simulink model "asynchronous_model"  (R2020a)
settings: Solver=FixedStepAuto  StartTime=0.0  StopTime=50  FixedStep=0.01  MaxStep=.001  RelTol=1e-3
values from neighbouring files (symbols this model uses):
  C_viscous = 0    [load_system_param.m]    (also in run_one_simulation.m = sys_param('C_viscous'); run_simulation.m = sys_param('C_viscous'))
  Gamma = 0.00107    [load_system_param.m]    (also in run_one_simulation.m = sys_param('Gamma'); run_simulation.m = sys_param('Gamma'))
  Inertia = 0.0023    [load_system_param.m]    (also in run_one_simulation.m = sys_param('I'); run_simulation.m = sys_param('I'))
  K = 0.525    [load_system_param.m]    (also in run_one_simulation.m = sys_param('K'); run_simulation.m = sys_param('K'))
  K_muscle = 0    [load_system_param.m]    (also in run_one_simulation.m = sys_param('K_muscle'); run_simulation.m = sys_param('K_muscle'))
  SA_kernel = asynch_gain * gain_constant * (1 - K_r) * temp_kernel    [run_one_simulation.m]    (also in run_simulation.m = asynch_gain * gain_constant * (1 - synch_gain_range(k)) * te)
  synch_gain = K_r * gain_constant    [run_one_simulation.m]    (also in run_simulation.m = synch_gain_range(k) * gain_constant)
  v_initial = 0    [load_system_param.m]    (also in run_one_simulation.m = sys_param('v_initial'); run_simulation.m = sys_param('v_initial'))
  x_initial = 0.1    [load_system_param.m]    (also in run_one_simulation.m = sys_param('x_initial'); run_simulation.m = sys_param('x_initial'))
undefined symbols (not defined in the file or in its folder): synch_w
settings Model: OrderedModelArguments=off  Creator=nickgravish  LastModifiedBy=Administrator
settings DataIOCC: ReturnWorkspaceOutputs=off
settings DebuggingCC: ArithmeticOperatorsInVariantConditions=warning
settings SFSimCC: SimUseLocalCustomCode=off  CustomCodeUndefinedFunction=UseInterfaceOnly
settings RTWCC: RTWUseLocalCustomCode=off
settings CodeAppCC: StateflowObjectComments=on
settings SimscapeCC: SimscapeNormalizeSystem=off

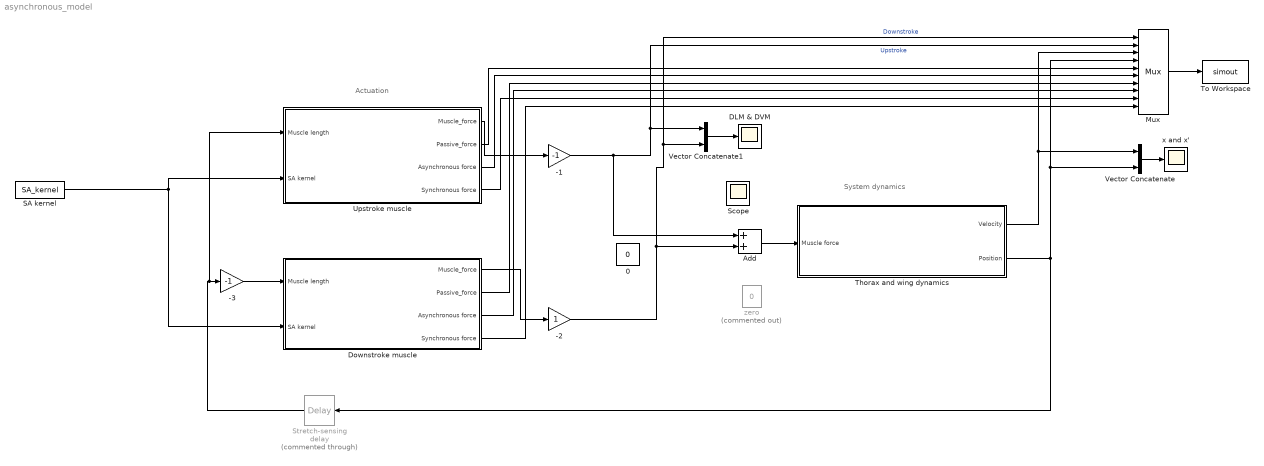
== system asynchronous_model ==
  note: Actuation
  note: System dynamics
  -1 : Gain  Gain=-1
  -2 : Gain
  -3 : Gain  Gain=-1
  Add : Sum
  DLM & DVM : Scope
  Downstroke muscle : Subsystem
  Mux : Mux  Inputs=10
  SA kernel : Constant  Value=SA_kernel
  Stretch-sensing delay : TransportDelay  Commented=through  DelayTime=0
  Thorax and wing dynamics : Subsystem
  To Workspace : ToWorkspace  VariableName=simout  SaveFormat=Timeseries  SampleTime=-1
  Upstroke muscle : Subsystem
  Vector Concatenate : Concatenate
  Vector Concatenate1 : Concatenate
  x and x' : Scope
  zero : Constant  Commented=on  Value=0
  0 : Constant  IOType=siggen  Value=0
  Scope : Scope
  wires:
  Vector Concatenate/1 -> x and x'/1
  -2/1 -> Add/2, Mux/1, Vector Concatenate1/2  "Downstroke"
  -1/1 -> Mux/2, Vector Concatenate1/1, Add/1  "Upstroke"
  Vector Concatenate1/1 -> DLM & DVM/1
  Mux/1 -> To Workspace/1
  Downstroke muscle/1(Muscle_force) -> -2/1
  Thorax and wing dynamics/1(Velocity) -> Mux/3, Vector Concatenate/1
  Thorax and wing dynamics/2(Position) -> Vector Concatenate/2, Mux/4, Stretch-sensing delay/1
  Upstroke muscle/1(Muscle_force) -> -1/1
  Stretch-sensing delay/1 -> Upstroke muscle/1(Muscle length), -3/1
  SA kernel/1 -> Upstroke muscle/2(SA kernel), Downstroke muscle/2(SA kernel)
  -3/1 -> Downstroke muscle/1(Muscle length)
  Downstroke muscle/3(Asynchronous force) -> Mux/8
  Downstroke muscle/2(Passive_force) -> Mux/7
  Upstroke muscle/3(Asynchronous force) -> Mux/6
  Upstroke muscle/2(Passive_force) -> Mux/5
  Add/1 -> Thorax and wing dynamics/1(Muscle force)
  Upstroke muscle/4(Synchronous force) -> Mux/9
  Downstroke muscle/4(Synchronous force) -> Mux/10

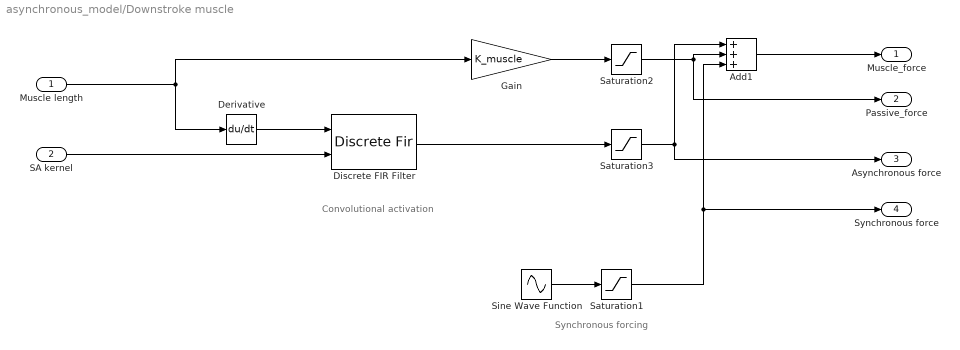
== system asynchronous_model/Downstroke muscle ==
  note: Convolutional activation
  note: Synchronous forcing
  Muscle length : Inport
  SA kernel : Inport  Port=2
  Add1 : Sum  Inputs=+++
  Derivative : Derivative
  Discrete FIR Filter : DiscreteFir  CoefSource=Input port  Coefficients=[0, 0, 2]  InputProcessing=Columns as channels (frame based)
      settings: InputPortMap=u0,u1
  Gain : Gain  Gain=K_muscle
  Saturation1 : Saturate  UpperLimit=Inf  LowerLimit=0
  Saturation2 : Saturate  UpperLimit=Inf  LowerLimit=0
  Saturation3 : Saturate  UpperLimit=Inf  LowerLimit=0
  Sine Wave Function : Sin  Amplitude=synch_gain  Frequency=synch_w  Phase=pi  SampleTime=0
  Muscle_force : Outport
  Passive_force : Outport  Port=2
  Asynchronous force : Outport  Port=3
  Synchronous force : Outport  Port=4
  wires:
  SA kernel/1 -> Discrete FIR Filter/2
  Add1/1 -> Muscle_force/1
  Gain/1 -> Saturation2/1
  Muscle length/1 -> Gain/1, Derivative/1
  Saturation2/1 -> Add1/2, Passive_force/1
  Saturation3/1 -> Add1/1, Asynchronous force/1
  Derivative/1 -> Discrete FIR Filter/1
  Discrete FIR Filter/1 -> Saturation3/1
  Saturation1/1 -> Synchronous force/1, Add1/3
  Sine Wave Function/1 -> Saturation1/1

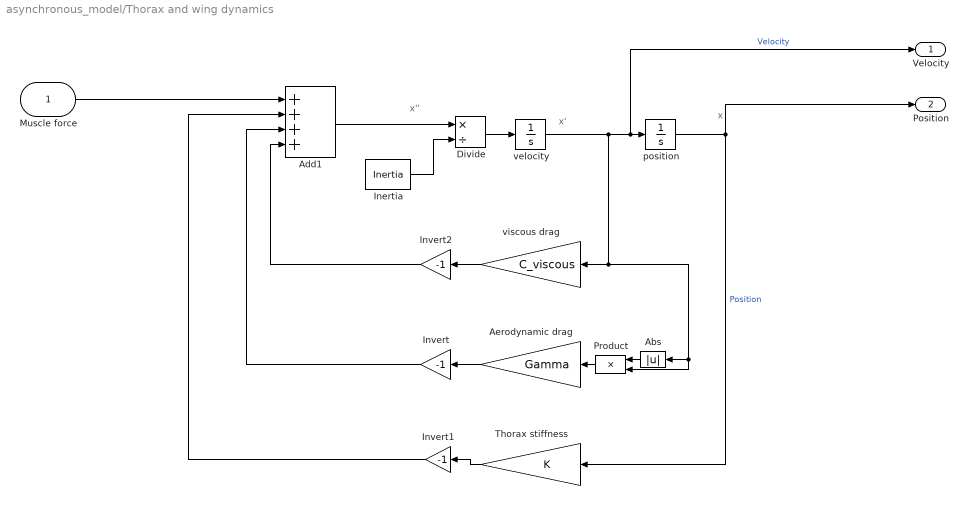
== system asynchronous_model/Thorax and wing dynamics ==
  note: x
  note: x''
  note: x'
  Muscle force : Inport
  Abs : Abs
  Add1 : Sum  Inputs=++++
  Aerodynamic drag : Gain  Gain=Gamma
  Divide : Product  Inputs=*/
  Inertia : Constant  Value=Inertia
  Invert : Gain  Gain=-1
  Invert1 : Gain  Gain=-1
  Invert2 : Gain  Gain=-1
  Product : Product
  Thorax stiffness : Gain  Gain=K
  position : Integrator  InitialCondition=x_initial  ContinuousStateAttributes='Position'
  velocity : Integrator  InitialCondition=v_initial  ContinuousStateAttributes='Velocity'
  viscous drag : Gain  Gain=C_viscous
  Velocity : Outport
  Position : Outport  Port=2
  wires:
  Aerodynamic drag/1 -> Invert/1
  Thorax stiffness/1 -> Invert1/1
  Divide/1 -> velocity/1
  Add1/1 -> Divide/1
  Muscle force/1 -> Add1/1
  velocity/1 -> Product/2, Abs/1, viscous drag/1, Velocity/1, position/1  "Velocity"
  viscous drag/1 -> Invert2/1
  Inertia/1 -> Divide/2
  position/1 -> Thorax stiffness/1, Position/1  "Position"
  Invert2/1 -> Add1/4
  Abs/1 -> Product/1
  Product/1 -> Aerodynamic drag/1
  Invert/1 -> Add1/3
  Invert1/1 -> Add1/2

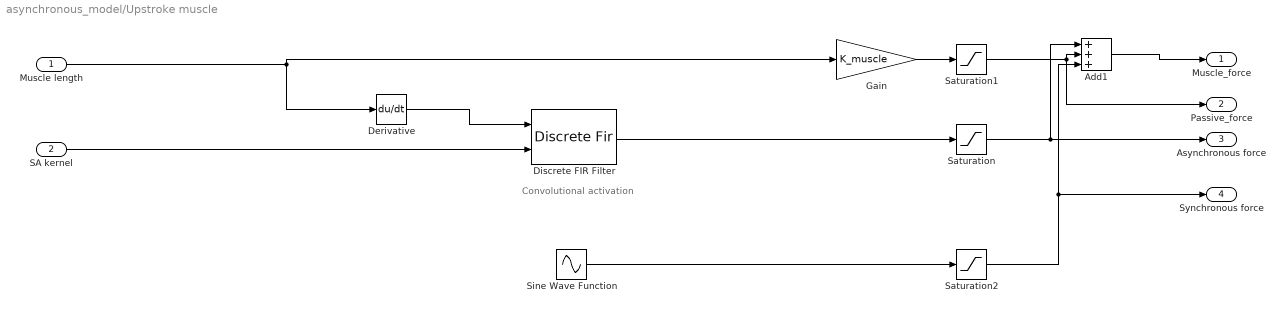
== system asynchronous_model/Upstroke muscle ==
  note: Convolutional activation
  Muscle length : Inport
  SA kernel : Inport  Port=2
  Add1 : Sum  Inputs=+++
  Derivative : Derivative
  Discrete FIR Filter : DiscreteFir  CoefSource=Input port  Coefficients=[0, 0, 2]  InputProcessing=Columns as channels (frame based)
      settings: InputPortMap=u0,u1
  Gain : Gain  Gain=K_muscle
  Saturation : Saturate  UpperLimit=Inf  LowerLimit=0
  Saturation1 : Saturate  UpperLimit=Inf  LowerLimit=0
  Saturation2 : Saturate  UpperLimit=Inf  LowerLimit=0
  Sine Wave Function : Sin  Amplitude=synch_gain  Frequency=synch_w  SampleTime=0
  Muscle_force : Outport
  Passive_force : Outport  Port=2
  Asynchronous force : Outport  Port=3
  Synchronous force : Outport  Port=4
  wires:
  Gain/1 -> Saturation1/1
  Saturation/1 -> Asynchronous force/1, Add1/1
  Muscle length/1 -> Derivative/1, Gain/1
  SA kernel/1 -> Discrete FIR Filter/2
  Add1/1 -> Muscle_force/1
  Saturation1/1 -> Passive_force/1, Add1/2
  Discrete FIR Filter/1 -> Saturation/1
  Derivative/1 -> Discrete FIR Filter/1
  Sine Wave Function/1 -> Saturation2/1
  Saturation2/1 -> Synchronous force/1, Add1/3
